simulink model "NoFricModel"  (R2024a)
settings: Solver=ode15s  StartTime=0.0  StopTime=2  RelTol=1e-3
values from neighbouring files (symbols this model uses):
  Achsabstand = 0.15    [Model1Sensibilities.m]    (also in Model1numericalPSA.m; Model2Sensibilities.m; Modellvalidierung.m; MotorSens2.m)
  Reifen_Radius = 0.04    [Model1Sensibilities.m]    (also in Model1numericalPSA.m; Model2Sensibilities.m; Modellvalidierung.m; MotorSens2.m)
  StartPos = [0.3;0.3]    [Model1Sensibilities.m]    (also in Model1numericalPSA.m; Model2Sensibilities.m; MotorSens2.m; Motor_Sensitivitaet.m)
libraries: mobileRoboticsLib x1
settings Model: Creator=Jakob Reindl  LastModifiedBy=jakob

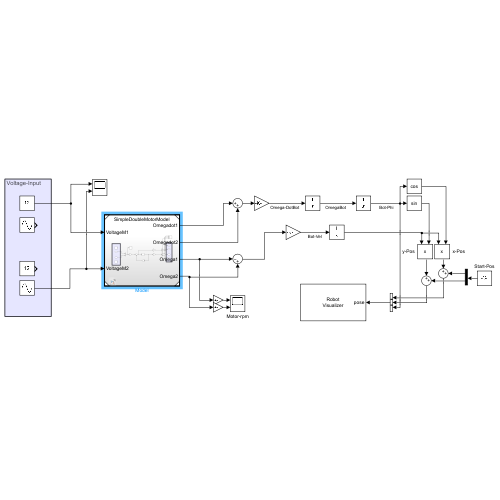
[thumbnail: Simulink's stored preview of the top-level diagram]
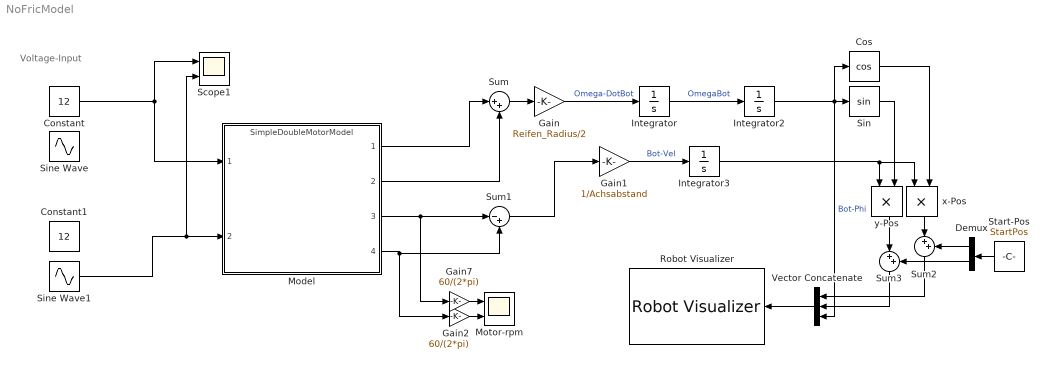
== system NoFricModel ==
  note: Voltage-Input
  Constant : Constant  Value=12  SampleTime=1
  Constant1 : Constant  Value=12  SampleTime=1
  Cos : Trigonometry  Operator=cos
  Demux : Demux  Outputs=2
  Gain : Gain  Gain=Reifen_Radius/2
  Gain1 : Gain  Gain=1/Achsabstand
  Gain2 : Gain  Gain=60/(2*pi)
  Gain7 : Gain  Gain=60/(2*pi)
  Integrator : Integrator
  Integrator2 : Integrator
  Integrator3 : Integrator
  Model : ModelReference  ModelNameDialog=SimpleDoubleMotorModel.slx  SimulationMode=Normal  ModelReferenceVersion=1.3
  Motor-rpm : Scope  NumInputPorts=2
  Robot Visualizer : mobileRoboticsLib/Environments/Robot Visualizer  robotRadius=0.1  mapName=myMap  showTrajectory=on  hasWaypoints=off  hasLidar=off  sensorOffset=[ 0, 0 ]  scanAngles=[ -pi/4, 0, pi/4 ]  hasObjDetector=off  objDetectorOffset=[ 0, 0 ]  objDetectorAngle=0  objDetectorFOV=pi/4  objDetectorMaxRange=5  objectColors=[ 1, 0, 0; 0, 1, 0; 0, 0, 1 ]  objectMarkers=s
  Scope1 : Scope  NumInputPorts=2
  Sin : Trigonometry
  Sine Wave : Sin  Amplitude=4  Bias=8  Frequency=2  SampleTime=0
  Sine Wave1 : Sin  Amplitude=2  Bias=9  Frequency=8  SampleTime=0
  Start-Pos : Constant  Value=StartPos
  Sum : Sum  Inputs=|++
  Sum1 : Sum  Inputs=|-+
  Sum2 : Sum  Inputs=|++
  Sum3 : Sum  Inputs=|++
  Vector Concatenate : Concatenate  NumInputs=3
  x-Pos : Product
  y-Pos : Product
  wires:
  Constant/1 -> Model/1, Scope1/1
  Model/1 -> Sum/1
  Model/2 -> Sum/2
  Sum/1 -> Gain/1
  Sum1/1 -> Gain1/1
  Gain/1 -> Integrator/1  "Omega-DotBot"
  Integrator/1 -> Integrator2/1  "OmegaBot"
  Gain1/1 -> Integrator3/1  "Bot-Vel"
  Integrator2/1 -> Cos/1, Vector Concatenate/3, Sin/1  "Bot-Phi"
  Integrator3/1 -> x-Pos/1, y-Pos/1
  Cos/1 -> x-Pos/2
  Sin/1 -> y-Pos/2
  x-Pos/1 -> Sum2/1
  Vector Concatenate/1 -> Robot Visualizer/1
  Model/3 -> Gain7/1, Sum1/1
  Model/4 -> Gain2/1, Sum1/2
  Demux/1 -> Sum2/2
  y-Pos/1 -> Sum3/1
  Sum2/1 -> Vector Concatenate/1
  Start-Pos/1 -> Demux/1
  Demux/2 -> Sum3/2
  Sum3/1 -> Vector Concatenate/2
  Gain7/1 -> Motor-rpm/1
  Gain2/1 -> Motor-rpm/2
  Sine Wave1/1 -> Scope1/2, Model/2
